simulink model "Ej3"  (R2018a)
settings: Solver=VariableStepAuto  StartTime=0.0  StopTime=100  RelTol=1e-3
values from neighbouring files (symbols this model uses):
  a = 200    [Ej1_params.m]    (also in Ej2_params.m; Ej3_params.m; Ej4_params.m)
  b = 10000    [Ej1_params.m]    (also in Ej2_params.m; Ej3_params.m; Ej4_params.m)
  g = 9.82    [Ej1_params.m]    (also in Ej2_params.m; Ej3_params.m; Ej4_params.m)
  ki = .1    (= 0.1)    [Ej3_params.m]    (also in Ej4_params.m = double(subs(ki_solu, [m_s, a_s, b_s, p_place_s], [m, a, b, p)
  kp = 1    [Ej3_params.m]    (also in Ej4_params.m = double(subs(kp_solu, [m_s, a_s, b_s, p_place_s], [m, a, b, p)
  m = 1500    [Ej1_params.m]    (also in Ej2_params.m = 1000; Ej3_params.m = 1000; Ej4_params.m = 1000)
settings Model: Creator=joses  LastModifiedBy=joses

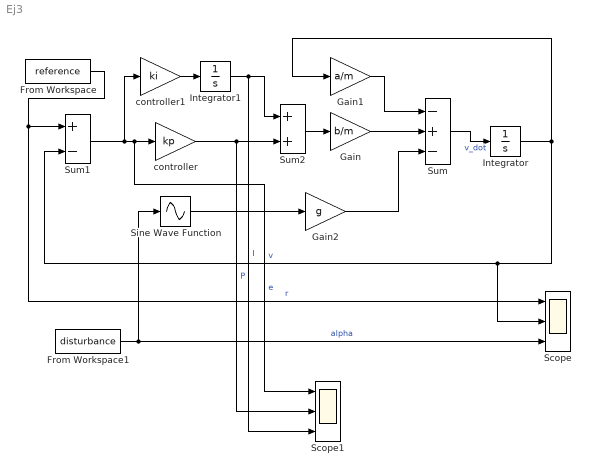
== system Ej3 ==
  From Workspace : FromWorkspace  VariableName=reference  SampleTime=.01
  From Workspace1 : FromWorkspace  VariableName=disturbance  SampleTime=.01
  Gain : Gain  Gain=b/m
  Gain1 : Gain  Gain=a/m
  Gain2 : Gain  Gain=g
  Integrator : Integrator
  Integrator1 : Integrator
  Scope : Scope  NumInputPorts=3
  Scope1 : Scope  NumInputPorts=3
  Sine Wave Function : Sin  TimeSource=Use external signal  SampleTime=0
  Sum : Sum  Inputs=-+-
  Sum1 : Sum  Inputs=+-
  Sum2 : Sum
  controller : Gain  Gain=kp
  controller1 : Gain  Gain=ki
  wires:
  Sum/1 -> Integrator/1  "v_dot"
  Gain/1 -> Sum/2
  Gain1/1 -> Sum/1
  Integrator/1 -> Sum1/2, Scope/2, Gain1/1  "v"
  From Workspace/1 -> Sum1/1, Scope/1  "r"
  Sine Wave Function/1 -> Gain2/1
  From Workspace1/1 -> Sine Wave Function/1, Scope/3  "alpha"
  Gain2/1 -> Sum/3
  Sum1/1 -> controller1/1, Scope1/1, controller/1  "e"
  controller/1 -> Scope1/2, Sum2/2  "P"
  controller1/1 -> Integrator1/1
  Integrator1/1 -> Scope1/3, Sum2/1  "I"
  Sum2/1 -> Gain/1
